simulink model "Airplane_simulator"  (R2023b)
settings: Solver=ode4  StartTime=0  StopTime=tfinal  FixedStep=dt  RelTol=1e-3
values from neighbouring files (symbols this model uses):
  delta_control = [deg2rad([delta_aileron, delta_rudder, delta_elevator]), delta_thrust]    [main_code.m]
  F_gravity_0 = mass * gravity * [sin(states_0(8));                                 -cos(states_0(8)) * sin(states_0(7));                                 -cos(states_0(8)) * cos(states_0(7))]    [main_code.m]
  gravity = aircraft_data(52)    [main_code.m]
  Ixx = aircraft_data(53)    [main_code.m]
  Iyy = aircraft_data(54)    [main_code.m]
  Izz = aircraft_data(55)    [main_code.m]
  M_0 = [0; 0; 0]    [main_code.m]
  mass = aircraft_data(51)    [main_code.m]
  Matrix_controls = [0, Xde, Xdth, 0 ... (first row only)    [main_code.m]
  Matrix_states = [Xu, 0, Xw, 0, 0, 0, 0 ... (first row only)    [main_code.m]
  p0 = states_0(4)    [main_code.m]
  phi0 = states_0(7)    [main_code.m]
  psi0 = states_0(9)    [main_code.m]
  q0 = states_0(5)    [main_code.m]
  r0 = states_0(6)    [main_code.m]
  states_0 = aircraft_data(4:15)    [main_code.m]
  theta0 = states_0(8)    [main_code.m]
  u0 = states_0(1)    [main_code.m]
  v0 = states_0(2)    [main_code.m]
  w0 = states_0(3)    [main_code.m]
  x0 = states_0(10)    [main_code.m]
  y0 = states_0(11)    [main_code.m]
  z0 = states_0(12)    [main_code.m]
libraries: simulink_extras x6, shared6dof x1, aerolibasang x1, dspsigops x1
settings Model: Creator=Ahmed Raamadan  LastModifiedBy=Ahmed Raamadan

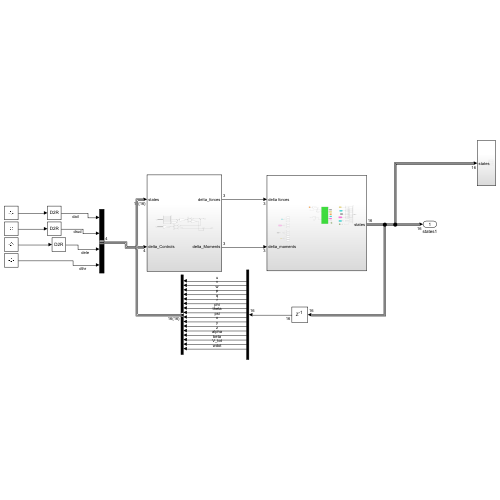
[thumbnail: Simulink's stored preview of the top-level diagram]
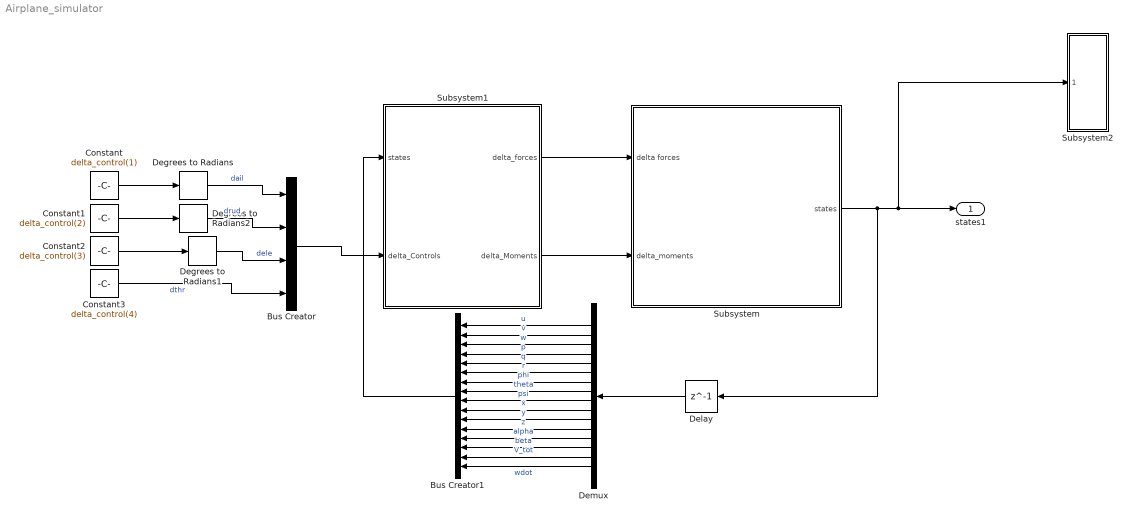
== system Airplane_simulator ==
  Bus Creator : BusCreator  Inputs=4
  Bus Creator1 : BusCreator  Inputs=16
  Constant : Constant  Value=delta_control(1)
  Constant1 : Constant  Value=delta_control(2)
  Constant2 : Constant  Value=delta_control(3)
  Constant3 : Constant  Value=delta_control(4)
  Degrees to Radians : simulink_extras/Transformations/Degrees to Radians
  Degrees to Radians1 : simulink_extras/Transformations/Degrees to Radians
  Degrees to Radians2 : simulink_extras/Transformations/Degrees to Radians
  Delay : Delay  DelayLength=1  InitialCondition=[states_0;0;0;0;0]
  Demux : Demux  Outputs=16
  Subsystem : Subsystem
  Subsystem1 : Subsystem
  Subsystem2 : Subsystem
  states1 : Outport
  wires:
  Subsystem1/1(delta_forces) -> Subsystem/1(delta forces)
  Subsystem1/2(delta_Moments) -> Subsystem/2(delta_moments)
  Bus Creator/1 -> Subsystem1/2(delta_Controls)
  Constant/1 -> Degrees to Radians/1
  Degrees to Radians/1 -> Bus Creator/1  "dail"
  Constant1/1 -> Degrees to Radians2/1
  Degrees to Radians2/1 -> Bus Creator/2  "drud"
  Constant3/1 -> Bus Creator/4  "dthr"
  Constant2/1 -> Degrees to Radians1/1
  Subsystem/1(states) -> states1/1, Subsystem2/1(states), Delay/1
  Bus Creator1/1 -> Subsystem1/1(states)
  Demux/1 -> Bus Creator1/1  "u"
  Demux/2 -> Bus Creator1/2  "v"
  Demux/3 -> Bus Creator1/3  "w"
  Demux/4 -> Bus Creator1/4  "p"
  Demux/5 -> Bus Creator1/5  "q"
  Demux/6 -> Bus Creator1/6  "r"
  Demux/7 -> Bus Creator1/7  "phi"
  Demux/8 -> Bus Creator1/8  "theta"
  Demux/9 -> Bus Creator1/9  "psi"
  Demux/10 -> Bus Creator1/10  "x"
  Demux/11 -> Bus Creator1/11  "y"
  Demux/12 -> Bus Creator1/12  "z"
  Demux/13 -> Bus Creator1/13  "alpha"
  Demux/14 -> Bus Creator1/14  "beta"
  Demux/15 -> Bus Creator1/15  "V_tot"
  Demux/16 -> Bus Creator1/16  "wdot"
  Delay/1 -> Demux/1
  Degrees to Radians1/1 -> Bus Creator/3  "dele"

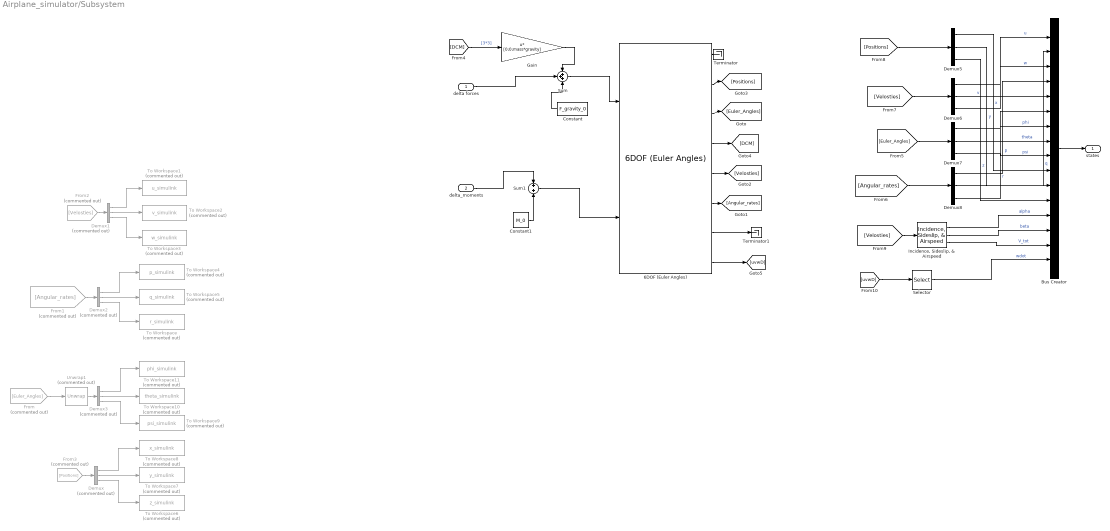
== system Airplane_simulator/Subsystem ==
  delta forces : Inport
  delta_moments : Inport  Port=2
  6DOF (Euler Angles) : shared6dof/6DOF (Euler Angles)  units=English (Velocity in ft/s)  mtype=Fixed  rep=Euler Angles  xme_0=[x0 y0 z0]  Vm_0=[u0 v0 w0]  eul_0=[phi0 theta0 psi0]  pm_0=[p0 q0 r0]  mass_0=mass  mass_e=0.5  mass_f=2.0  inertia=Inertia  inertia_e=eye(3)  inertia_f=2*eye(3)  k_quat=1.0  vre_flag=on  abi_flag=off  aMode=0  xme_statename=''  Vm_statename=''  eul_statename=''  quat_statename=''  pm_statename=''  mass_statename=''
  Bus Creator : BusCreator  Inputs=16
  Constant : Constant  Value=F_gravity_0
  Constant1 : Constant  Value=M_0
  Demux{,1..3} (4 alike) : Demux  Commented=on  Outputs=3
  Demux{5..8} (4 alike) : Demux  Outputs=3
  From : From  Commented=on  GotoTag=Euler_Angles
  From1 : From  Commented=on  GotoTag=Angular_rates
  From2 : From  Commented=on  GotoTag=Velosties
  From3 : From  Commented=on  GotoTag=Positions
  Gain : Gain  Gain=[0;0;mass*gravity]  Multiplication=Matrix(u*K)
  "Incidence, Sideslip, & Airspeed" : aerolibasang/Incidence, Sideslip, & Airspeed
  Selector : Selector  InputPortWidth=3  IndexOptions=Index vector (dialog)  Indices=[3]  OutputSizes=1
  Sum : Sum  Inputs=+++
  Sum1 : Sum
  Terminator : Terminator
  Terminator1 : Terminator
  To Workspace : ToWorkspace  Commented=on  VariableName=r_simulink  SaveFormat=Timeseries  SampleTime=-1
  To Workspace1 : ToWorkspace  Commented=on  VariableName=u_simulink  SaveFormat=Timeseries  SampleTime=-1
  To Workspace10 : ToWorkspace  Commented=on  VariableName=theta_simulink  SaveFormat=Timeseries  SampleTime=-1
  To Workspace11 : ToWorkspace  Commented=on  VariableName=phi_simulink  SaveFormat=Timeseries  SampleTime=-1
  To Workspace2 : ToWorkspace  Commented=on  VariableName=v_simulink  SaveFormat=Timeseries  SampleTime=-1
  To Workspace3 : ToWorkspace  Commented=on  VariableName=w_simulink  SaveFormat=Timeseries  SampleTime=-1
  To Workspace4 : ToWorkspace  Commented=on  VariableName=p_simulink  SaveFormat=Timeseries  SampleTime=-1
  To Workspace5 : ToWorkspace  Commented=on  VariableName=q_simulink  SaveFormat=Timeseries  SampleTime=-1
  To Workspace6 : ToWorkspace  Commented=on  VariableName=z_simulink  SaveFormat=Timeseries  SampleTime=-1
  To Workspace7 : ToWorkspace  Commented=on  VariableName=y_simulink  SaveFormat=Timeseries  SampleTime=-1
  To Workspace8 : ToWorkspace  Commented=on  VariableName=x_simulink  SaveFormat=Timeseries  SampleTime=-1
  To Workspace9 : ToWorkspace  Commented=on  VariableName=psi_simulink  SaveFormat=Timeseries  SampleTime=-1
  Unwrap1 : dspsigops/Unwrap  Commented=on  tol=pi  running=off
  states : Outport
  wires:
  Unwrap1/1 -> Demux3/1
  delta forces/1 -> Sum/2
  Demux3/2 -> To Workspace10/1
  "Incidence, Sideslip, & Airspeed"/3 -> Bus Creator/15  "V_tot"
  Demux/1 -> To Workspace8/1
  6DOF (Euler Angles)/3 -> [Euler_Angles]
  Demux1/2 -> To Workspace2/1
  Demux8/1 -> Bus Creator/4  "p"
  Demux1/1 -> To Workspace1/1
  Demux7/1 -> Bus Creator/7  "phi"
  [DCM] -> Gain/1  "[3*3]"
  Demux2/3 -> To Workspace/1
  Demux/3 -> To Workspace6/1
  [Velosties] -> "Incidence, Sideslip, & Airspeed"/1
  Demux3/1 -> To Workspace11/1
  6DOF (Euler Angles)/1 -> Terminator/1
  6DOF (Euler Angles)/8 -> [uvwD]
  [Positions] -> Demux5/1
  Demux6/1 -> Bus Creator/1  "u"
  Demux8/2 -> Bus Creator/5  "q"
  From2/1 -> Demux1/1
  6DOF (Euler Angles)/7 -> Terminator1/1
  Gain/1 -> Sum/1
  From1/1 -> Demux2/1
  Demux1/3 -> To Workspace3/1
  Demux6/2 -> Bus Creator/2  "v"
  Demux2/1 -> To Workspace4/1
  6DOF (Euler Angles)/2 -> [Positions]
  Demux2/2 -> To Workspace5/1
  [uvwD] -> Selector/1
  Demux5/3 -> Bus Creator/12  "z"
  6DOF (Euler Angles)/5 -> [Velosties]
  From3/1 -> Demux/1
  Demux6/3 -> Bus Creator/3  "w"
  Demux7/2 -> Bus Creator/8  "theta"
  Demux7/3 -> Bus Creator/9  "psi"
  Selector/1 -> Bus Creator/16  "wdot"
  Demux/2 -> To Workspace7/1
  Demux8/3 -> Bus Creator/6  "r"
  6DOF (Euler Angles)/6 -> [Angular_rates]
  From/1 -> Unwrap1/1
  Demux5/2 -> Bus Creator/11  "y"
  Constant1/1 -> Sum1/2
  Constant/1 -> Sum/3
  delta_moments/1 -> Sum1/1
  Demux5/1 -> Bus Creator/10  "x"
  6DOF (Euler Angles)/4 -> [DCM]
  Demux3/3 -> To Workspace9/1
  "Incidence, Sideslip, & Airspeed"/2 -> Bus Creator/14  "beta"
  Sum/1 -> 6DOF (Euler Angles)/1
  "Incidence, Sideslip, & Airspeed"/1 -> Bus Creator/13  "alpha"
  [Angular_rates] -> Demux8/1
  Sum1/1 -> 6DOF (Euler Angles)/2
  Bus Creator/1 -> states/1
  [Velosties] -> Demux6/1
  [Euler_Angles] -> Demux7/1

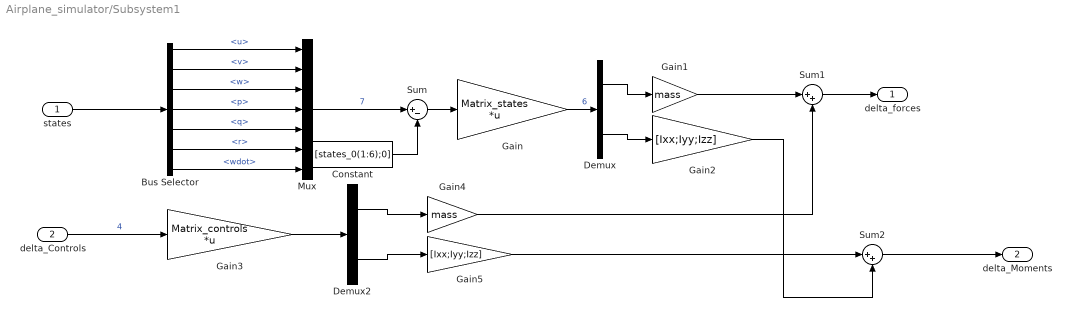
== system Airplane_simulator/Subsystem1 ==
  states : Inport
  delta_Controls : Inport  Port=2
  Bus Selector : BusSelector  OutputSignals=u,v,w,p,q,r,wdot
  Constant : Constant  Value=[states_0(1:6);0]  SampleTime=-1
  Demux : Demux  Outputs=2
  Demux2 : Demux  Outputs=2
  Gain : Gain  Gain=Matrix_states  Multiplication=Matrix(K*u)
  Gain1 : Gain  Gain=mass
  Gain2 : Gain  Gain=[Ixx;Iyy;Izz]
  Gain3 : Gain  Gain=Matrix_controls  Multiplication=Matrix(K*u)
  Gain4 : Gain  Gain=mass
  Gain5 : Gain  Gain=[Ixx;Iyy;Izz]
  Mux : Mux  Inputs=7
  Sum : Sum  Inputs=|+-
  Sum1 : Sum  Inputs=|++
  Sum2 : Sum  Inputs=|++
  delta_forces : Outport
  delta_Moments : Outport  Port=2
  wires:
  states/1 -> Bus Selector/1
  delta_Controls/1 -> Gain3/1  "4"
  Bus Selector/1 -> Mux/1  "<u>"
  Bus Selector/2 -> Mux/2  "<v>"
  Bus Selector/3 -> Mux/3  "<w>"
  Bus Selector/4 -> Mux/4  "<p>"
  Bus Selector/5 -> Mux/5  "<q>"
  Bus Selector/6 -> Mux/6  "<r>"
  Mux/1 -> Sum/1  "7"
  Bus Selector/7 -> Mux/7  "<wdot>"
  Gain1/1 -> Sum1/1
  Sum1/1 -> delta_forces/1
  Gain2/1 -> Sum2/2
  Sum2/1 -> delta_Moments/1
  Gain3/1 -> Demux2/1
  Demux2/2 -> Gain5/1
  Gain4/1 -> Sum1/2
  Gain5/1 -> Sum2/1
  Constant/1 -> Sum/2
  Gain/1 -> Demux/1  "6"
  Demux/1 -> Gain1/1
  Demux/2 -> Gain2/1
  Demux2/1 -> Gain4/1
  Sum/1 -> Gain/1

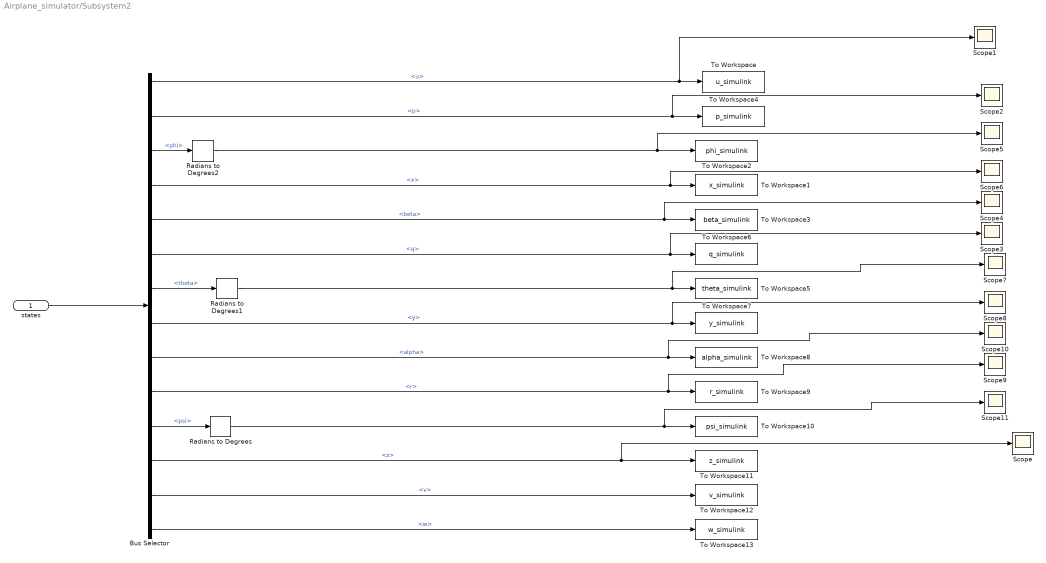
== system Airplane_simulator/Subsystem2 ==
  states : Inport
  Bus Selector : BusSelector  OutputSignals=u,p,phi,x,beta,q,theta,y,alpha,r,psi,z,v,w
  Radians to Degrees : simulink_extras/Transformations/Radians to Degrees
  Radians to Degrees1 : simulink_extras/Transformations/Radians to Degrees
  Radians to Degrees2 : simulink_extras/Transformations/Radians to Degrees
  Scope{,1..11} (12 alike) : Scope
  To Workspace : ToWorkspace  VariableName=u_simulink  SaveFormat=Timeseries  SampleTime=-1
  To Workspace1 : ToWorkspace  VariableName=x_simulink  SaveFormat=Timeseries  SampleTime=-1
  To Workspace10 : ToWorkspace  VariableName=psi_simulink  SaveFormat=Timeseries  SampleTime=-1
  To Workspace11 : ToWorkspace  VariableName=z_simulink  SaveFormat=Timeseries  SampleTime=-1
  To Workspace12 : ToWorkspace  VariableName=v_simulink  SaveFormat=Timeseries  SampleTime=-1
  To Workspace13 : ToWorkspace  VariableName=w_simulink  SaveFormat=Timeseries  SampleTime=-1
  To Workspace2 : ToWorkspace  VariableName=phi_simulink  SaveFormat=Timeseries  SampleTime=-1
  To Workspace3 : ToWorkspace  VariableName=beta_simulink  SaveFormat=Timeseries  SampleTime=-1
  To Workspace4 : ToWorkspace  VariableName=p_simulink  SaveFormat=Timeseries  SampleTime=-1
  To Workspace5 : ToWorkspace  VariableName=theta_simulink  SaveFormat=Timeseries  SampleTime=-1
  To Workspace6 : ToWorkspace  VariableName=q_simulink  SaveFormat=Timeseries  SampleTime=-1
  To Workspace7 : ToWorkspace  VariableName=y_simulink  SaveFormat=Timeseries  SampleTime=-1
  To Workspace8 : ToWorkspace  VariableName=alpha_simulink  SaveFormat=Timeseries  SampleTime=-1
  To Workspace9 : ToWorkspace  VariableName=r_simulink  SaveFormat=Timeseries  SampleTime=-1
  wires:
  Bus Selector/2 -> Scope2/1, To Workspace4/1  "<p>"
  states/1 -> Bus Selector/1
  Bus Selector/1 -> Scope1/1, To Workspace/1  "<u>"
  Bus Selector/3 -> Radians to Degrees2/1  "<phi>"
  Bus Selector/4 -> Scope6/1, To Workspace1/1  "<x>"
  Bus Selector/5 -> Scope4/1, To Workspace3/1  "<beta>"
  Bus Selector/6 -> Scope3/1, To Workspace6/1  "<q>"
  Bus Selector/7 -> Radians to Degrees1/1  "<theta>"
  Bus Selector/8 -> Scope8/1, To Workspace7/1  "<y>"
  Bus Selector/9 -> Scope10/1, To Workspace8/1  "<alpha>"
  Bus Selector/10 -> Scope9/1, To Workspace9/1  "<r>"
  Bus Selector/11 -> Radians to Degrees/1  "<psi>"
  Bus Selector/12 -> Scope/1, To Workspace11/1  "<z>"
  Bus Selector/13 -> To Workspace12/1  "<v>"
  Bus Selector/14 -> To Workspace13/1  "<w>"
  Radians to Degrees2/1 -> Scope5/1, To Workspace2/1
  Radians to Degrees1/1 -> Scope7/1, To Workspace5/1
  Radians to Degrees/1 -> Scope11/1, To Workspace10/1
